simulink model "State_Feedback_NON_Linear"  (R2022b)
settings: Solver=FixedStepAuto  StartTime=0.0  StopTime=10.0  FixedStep=step_size  RelTol=1e-3
undefined symbols (not defined in the file): a, theta_i, x_i, y_i, zeta
libraries: simulink_extras x2
settings Model: Creator=Musta  LastModifiedBy=Musta

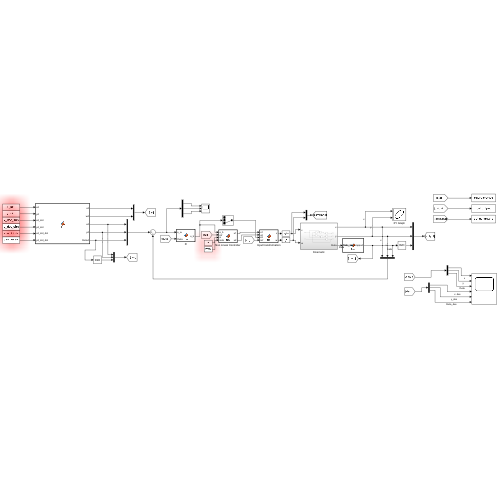
[thumbnail: Simulink's stored preview of the top-level diagram]
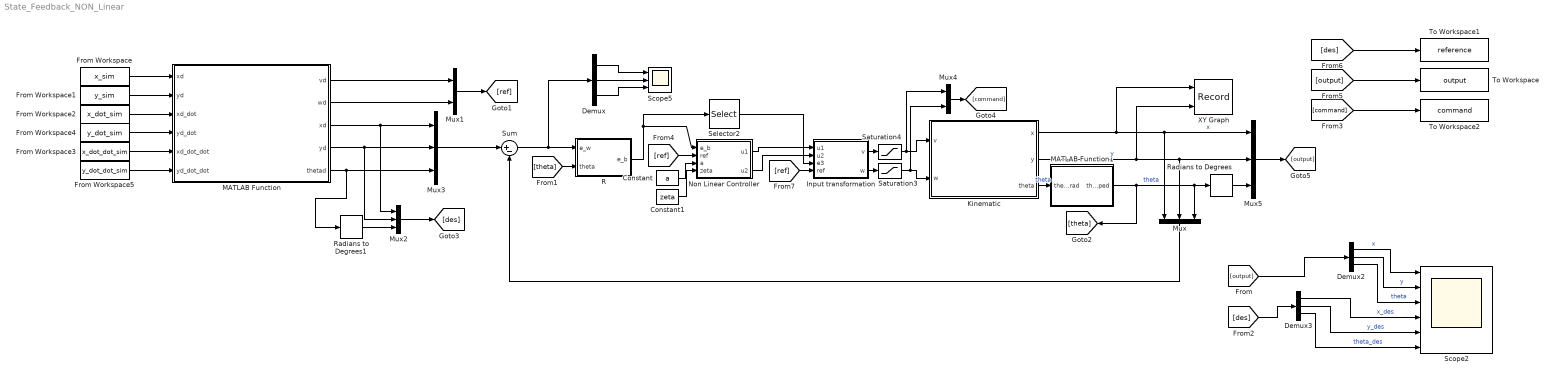
== system State_Feedback_NON_Linear ==
  Constant : Constant  Value=a
  Constant1 : Constant  Value=zeta
  Demux : Demux  Outputs=3
  Demux2 : Demux  Outputs=3
  Demux3 : Demux  Outputs=3
  From Workspace : FromWorkspace  VariableName=x_sim
  From Workspace1 : FromWorkspace  VariableName=y_sim
  From Workspace2 : FromWorkspace  VariableName=x_dot_sim
  From Workspace3 : FromWorkspace  VariableName=x_dot_dot_sim
  From Workspace4 : FromWorkspace  VariableName=y_dot_sim
  From Workspace5 : FromWorkspace  VariableName=y_dot_dot_sim
  Input transformation : MATLAB Function  TreatAsAtomicUnit=on
  Kinematic : Subsystem
  MATLAB Function : MATLAB Function  TreatAsAtomicUnit=on
  MATLAB Function1 : MATLAB Function  TreatAsAtomicUnit=on
  Mux{,2..3,5} (4 alike) : Mux  Inputs=3
  Mux1 : Mux  Inputs=2
  Mux4 : Mux  Inputs=2
  Non Linear Controller : MATLAB Function  TreatAsAtomicUnit=on
  R : MATLAB Function  TreatAsAtomicUnit=on
  Radians to Degrees : simulink_extras/Transformations/Radians to Degrees
  Radians to Degrees1 : simulink_extras/Transformations/Radians to Degrees
  Saturation3 : Saturate  UpperLimit=2  LowerLimit=-2
  Saturation4 : Saturate  UpperLimit=2  LowerLimit=-2
  Scope2 : Scope  NumInputPorts=6
  Scope5 : Scope  NumInputPorts=3
  Selector2 : Selector  InputPortWidth=3  IndexOptions=Index vector (dialog)  Indices=3  OutputSizes=1
  Sum : Sum  Inputs=|+-
  To Workspace : ToWorkspace  VariableName=output  SaveFormat=Structure With Time  SampleTime=-1
  To Workspace1 : ToWorkspace  VariableName=reference  SaveFormat=Structure With Time  SampleTime=-1
  To Workspace2 : ToWorkspace  VariableName=command  SaveFormat=Structure With Time  SampleTime=-1
  XY Graph : Record  FileSettingsInternal="{\"entries\":[{\"content\":{\"excelSettings\":{\"content\":{},\"type\":\"Streamout.ExcelSettings\"}},\"type\":\"Streamout.FileSettingStorage\",\"uuid\":\"682d1c13-c88e-46c2-b5c0-111468394261\"}],\"packageUris\":[\"http://schema.mathworks.com/mf0/streamout_blocks/R2020a\"],\"version\":\"1.0\"}"  Layout=[1 1]  SignalsInternal="{\"entries\":[{\"content\":{\"signals\":[{\"content\":{\"blockPath\":[\"State_Feedback_NON_Linear/XY Graph\"],\"channel\":[],\"dimensions\":[1],\"domain\":\"State_Feedback_NON_Linear/XY Graph\",\"lineColor\":\"#edb120\",\"plots\":[],\"port\":1,\"sid\":[],\"signalID\":100,\"signalName\":\"x\"},\"type\":\"RecordBlkView.Signal\",\"uuid\":\"26481353-9f29-4732-90e1-2d5a6569a59e\"},{\"content\":{\"blockPath\":[\"State_Feedback_NON_Linear/XY Graph\"],\"channel\":[],\"dimensions\":[1],\"domain\":\"State_Feedback_NON_Linear/XY Graph\",\"lineColor\":\"#7e2f8e\",\"plots\":[],\"port\":2,\"sid\":[],\"signalID\":103,\"signalName\":\"y\"},\"type\":\"RecordBlkView.Signal\",\"uuid\":\"55f820db-f055-4888-a435-fe00089df2d9\"}]},\"type\":\"RecordBlkView.InputSignals\",\"uuid\":\"cbe334b6-c6d3-4974-9fb9-82df0f4ac6dc\"}],\"packageUris\":[\"http://schema.mathworks.com/mf0/streamout_blocks/R2020a\"],\"version\":\"1.0\"}"  VisualizationBindings="{\"xyplotplugin\":{\"info\":[{\"series\":[],\"subplotID\":1}]}}"  CompatibilityTag=XY
  wires:
  Mux1/1 -> [ref]
  R/1(e_b) -> Non Linear Controller/1(e_b), Selector2/1
  From Workspace3/1 -> MATLAB Function/5(xd_dot_dot)
  From Workspace4/1 -> MATLAB Function/4(yd_dot)
  Constant1/1 -> Non Linear Controller/4(zeta)
  [ref] -> Input transformation/4(ref)
  From Workspace5/1 -> MATLAB Function/6(yd_dot_dot)
  MATLAB Function/5(thetad) -> Radians to Degrees1/1, Mux3/3
  Demux/2 -> Scope5/2
  MATLAB Function/2(wd) -> Mux1/2
  From Workspace1/1 -> MATLAB Function/2("yd ")
  Sum/1 -> R/1(e_w), Demux/1
  MATLAB Function/1(vd) -> Mux1/1
  Demux/1 -> Scope5/1
  MATLAB Function/3(xd) -> Mux2/1, Mux3/1
  Selector2/1 -> Input transformation/3(e3)
  [theta] -> R/2(theta)
  From Workspace/1 -> MATLAB Function/1("xd ")
  Mux2/1 -> [des]
  [ref] -> Non Linear Controller/2(ref)
  Constant/1 -> Non Linear Controller/3(a)
  MATLAB Function/4(yd) -> Mux2/2, Mux3/2
  Mux3/1 -> Sum/1
  Non Linear Controller/1(u1) -> Input transformation/1(u1)
  Non Linear Controller/2(u2) -> Input transformation/2(u2)
  Mux4/1 -> [command]
  Demux/3 -> Scope5/3
  From Workspace2/1 -> MATLAB Function/3(xd_dot)
  Input transformation/1(v) -> Saturation4/1
  Input transformation/2(w) -> Saturation3/1
  Saturation3/1 -> Mux4/2, Kinematic/2(w)
  Saturation4/1 -> Mux4/1, Kinematic/1(v)
  Radians to Degrees/1 -> Mux5/3
  Mux5/1 -> [output]
  Kinematic/1(x) -> XY Graph/1, Mux/1, Mux5/1  "x"
  Mux/1 -> Sum/2
  Demux2/1 -> Scope2/1  "x"
  Kinematic/2(y) -> XY Graph/2, Mux/2, Mux5/2  "y"
  [command] -> To Workspace2/1
  MATLAB Function1/1(theta_rad_wrapped) -> Mux/3, Radians to Degrees/1, [theta]  "theta"
  Demux3/3 -> Scope2/6  "theta_des"
  [output] -> To Workspace/1
  Demux2/3 -> Scope2/3  "theta"
  [des] -> Demux3/1
  [output] -> Demux2/1
  [des] -> To Workspace1/1
  Demux3/2 -> Scope2/5  "y_des"
  Demux2/2 -> Scope2/2  "y"
  Demux3/1 -> Scope2/4  "x_des"
  Kinematic/3(theta) -> MATLAB Function1/1(theta_rad)  "theta"
  Radians to Degrees1/1 -> Mux2/3

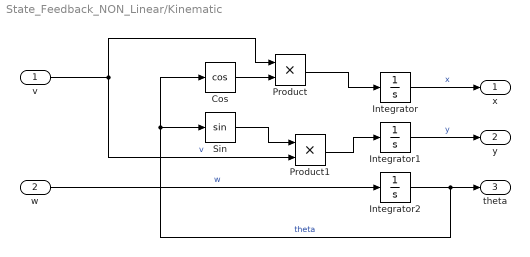
== system State_Feedback_NON_Linear/Kinematic ==
  v : Inport
  w : Inport  Port=2
  Cos : Trigonometry  Operator=cos
  Integrator : Integrator  InitialCondition=x_i
  Integrator1 : Integrator  InitialCondition=y_i
  Integrator2 : Integrator  InitialCondition=theta_i
  Product : Product
  Product1 : Product
  Sin : Trigonometry
  x : Outport
  y : Outport  Port=2
  theta : Outport  Port=3
  wires:
  w/1 -> Integrator2/1  "w"
  Product/1 -> Integrator/1
  v/1 -> Product/1, Product1/2  "v"
  Cos/1 -> Product/2
  Integrator1/1 -> y/1  "y"
  Integrator/1 -> x/1  "x"
  Integrator2/1 -> Cos/1, Sin/1, theta/1  "theta"
  Product1/1 -> Integrator1/1
  Sin/1 -> Product1/1

== matlab function State_Feedback_NON_Linear/MATLAB Function ==
  data: xd input; vd output; yd input; xd_dot input; yd_dot input; xd_dot_dot input; yd_dot_dot input; wd output; xd output; yd output; thetad output
function [vd, wd, xd, yd, thetad] = fcn(xd, yd, xd_dot, yd_dot, xd_dot_dot, yd_dot_dot)
    
    vd = sqrt(xd_dot.^2 + yd_dot.^2);
    wd = (xd_dot.*yd_dot_dot - xd_dot_dot.*yd_dot) / (xd_dot.^2 + yd_dot.^2);
    % thetad = atan2(yd_dot, xd_dot);
    thetad = mod(atan2(yd_dot,xd_dot), 2*pi);

    xd = xd;
    yd = yd;

end

== matlab function State_Feedback_NON_Linear/Non Linear Controller ==
  data: e_b input; u1 output; ref input; u2 output; a input; zeta input
function [u1,u2] = fcn(e_b, ref, a, zeta)

    b = (a^2 - ref(2)^2) / ref(1);

    k1 = 2*zeta*sqrt(b*ref(1) + ref(2)^2);
    k2 = b;
    k3 = 2*zeta*sqrt(b*ref(1) + ref(2)^2);

    u1 = -k1*e_b(1);
    u2 = (-k2*ref(1)*sin(e_b(3))*e_b(2)) / e_b(3)  -k3*e_b(3);

end

== matlab function State_Feedback_NON_Linear/Input transformation ==
  data: u1 input; v output; u2 input; e3 input; w output; ref input
function [v, w] = fcn(u1, u2, e3, ref)

    v = ref(1)*cos(e3) - u1;
    w = ref(2) - u2;

end

== matlab function State_Feedback_NON_Linear/MATLAB Function1 ==
  data: theta_rad input; theta_rad_wrapped output
function theta_rad_wrapped = fcn(theta_rad)

    if abs(theta_rad) < 5e-5
        theta_rad = 0;
    end

    theta_rad_wrapped = wrapTo2Pi(theta_rad);

end

== matlab function State_Feedback_NON_Linear/R ==
  data: e_w input; e_b output; theta input
function e_b  = fcn(e_w, theta)
    
    R = [cos(theta), sin(theta), 0;
        -sin(theta), cos(theta), 0;
         0, 0, 1];

    e_b = R * e_w;

end
